simulink model "model_with_initial_conditions_v1"  (R2024b)
settings: Solver=VariableStepAuto  StartTime=0.0  StopTime=10.0  RelTol=1e-3
undefined symbols (not defined in the file): K1, K2, m
settings Model: Creator=njpan  LastModifiedBy=jacksonwright

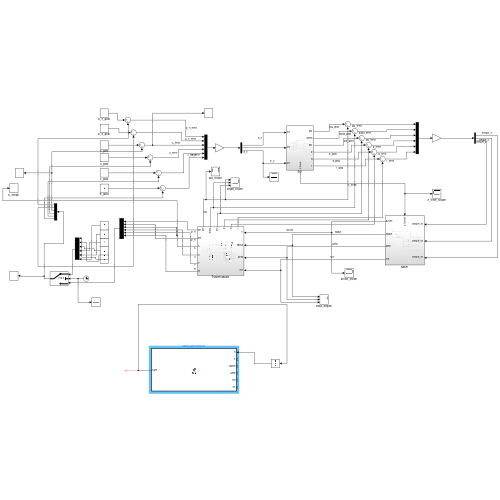
[thumbnail: Simulink's stored preview of the top-level diagram]
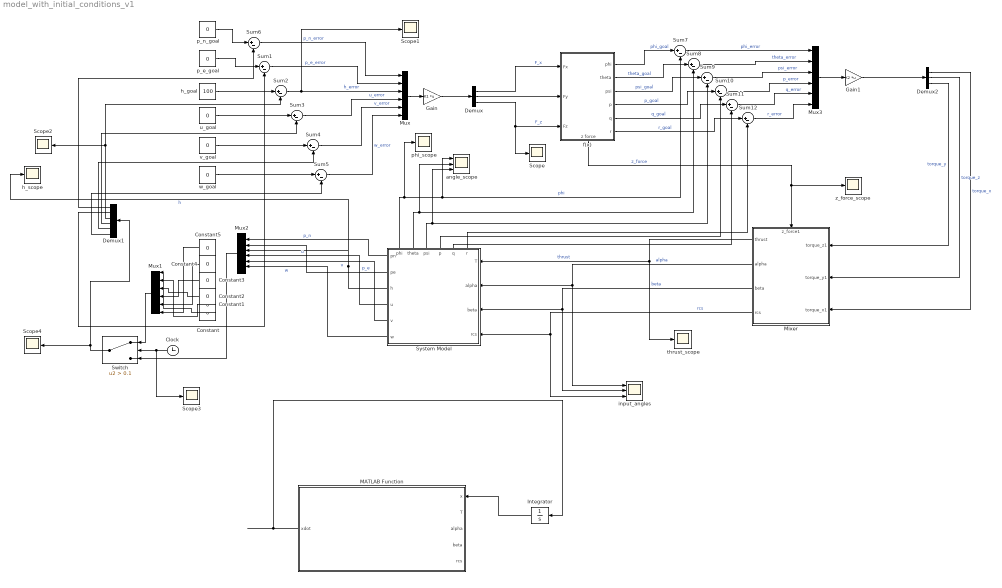
== system model_with_initial_conditions_v1 ==
  Clock : Clock
  Constant{,1..5} (6 alike) : Constant  Value=0
  Demux : Demux  Outputs=3
  Demux1 : Demux  Outputs=6
  Demux2 : Demux  Outputs=3
  Gain : Gain  Gain=K1  Multiplication=Matrix(K*u)
  Gain1 : Gain  Gain=K2  Multiplication=Matrix(K*u)
  Integrator : Integrator
  MATLAB Function : MATLAB Function  TreatAsAtomicUnit=on
  Mixer : Subsystem
      settings: PortSchema="{\"entries\":[{\"content\":{\"sides\":[{\"content\":{\"connectorIds\":[\"In1\",\"In2\",\"In3\"]},\"type\":\"ConnectorPlacement.EquallySpacedRectSide\",\"uuid\":\"e4ab6201-3171-425b-b678-f5a82ca77998\"},{\"content\":{\"connectorIds\":[\"Out1\",\"Out2\",\"Out3\",\"Out4\"],\"side\":\"RIGHT\"},\"type\":\"ConnectorPlacement.EquallySpacedRectSide\",\"uuid\":\"c6aae40c-8090-4a79-98d3-b60c0d3e66c5\"},{\"content\":{\"connectorIds\":[\"In4\"],\"side\":\"TOP\"},\"type\":\"ConnectorPlacement.EquallySpacedRectSide\",\"uuid\":\"89717ce5-f3d0-4b2e-8505-89723edf9773\"}]},\"type\":\"ConnectorPlacement.EquallySpacedConnector\",\"uuid\":\"ace876b5-bd23-4119-b1c7-2a296fd8fc0f\"}],\"packageUris\":[\"http://schema.mathworks.com/mf0/Connector/R2020b\"],\"version\":\"1.0\"}"
  Mux{,1..3} (4 alike) : Mux  Inputs=6
  Scope{,1..4} (5 alike) : Scope
  Sum{1..12} (12 alike) : Sum  Inputs=|+-
  Switch : Switch  Criteria=u2 > Threshold  Threshold=0.1  SaturateOnIntegerOverflow=off  InputSameDT=off
  System Model : Subsystem
      settings: PortSchema="{\"entries\":[{\"content\":{\"sides\":[{\"content\":{\"connectorIds\":[\"In1\",\"In2\",\"In3\",\"In4\"]},\"type\":\"ConnectorPlacement.EquallySpacedRectSide\",\"uuid\":\"8f145699-554a-4db3-b510-041d1b7c630e\"},{\"content\":{\"connectorIds\":[\"Out1\",\"Out2\",\"Out3\",\"Out4\",\"Out5\",\"Out6\"],\"side\":\"RIGHT\"},\"type\":\"ConnectorPlacement.EquallySpacedRectSide\",\"uuid\":\"6b085f61-d2ca-4739-902a-7b977a4f8bfa\"},{\"content\":{\"connectorIds\":[\"Out7\",\"Out8\",\"Out9\",\"Out10\",\"Out11\",\"Out12\"],\"side\":\"TOP\"},\"type\":\"ConnectorPlacement.EquallySpacedRectSide\",\"uuid\":\"4e3fe6dd-78f0-4e47-82e4-cad48dcfb91c\"}]},\"type\":\"ConnectorPlacement.EquallySpacedConnector\",\"uuid\":\"c7b0161a-0fea-43dd-8cee-87680deb6224\"}],\"packageUris\":[\"http://schema.mathworks.com/mf0/Connector/R2020b\"],\"version\":\"1.0\"}"
  angle_scope : Scope  NumInputPorts=3
  f(x) : Subsystem
      settings: PortSchema="{\"entries\":[{\"content\":{\"sides\":[{\"content\":{\"connectorIds\":[\"In1\",\"In2\",\"In3\"]},\"type\":\"ConnectorPlacement.EquallySpacedRectSide\",\"uuid\":\"e7aeffbb-634f-4153-9868-9d3e2e4280ad\"},{\"content\":{\"connectorIds\":[\"Out1\",\"Out2\",\"Out3\",\"Out4\",\"Out5\",\"Out6\"],\"side\":\"RIGHT\"},\"type\":\"ConnectorPlacement.EquallySpacedRectSide\",\"uuid\":\"e6d97028-2a10-4268-a5e2-55bbdc39a0c5\"},{\"content\":{\"side\":\"TOP\"},\"type\":\"ConnectorPlacement.EquallySpacedRectSide\",\"uuid\":\"fa716bc0-4a18-4661-a72d-62488d70bdc1\"},{\"content\":{\"connectorIds\":[\"Out7\"],\"side\":\"BOTTOM\"},\"type\":\"ConnectorPlacement.EquallySpacedRectSide\",\"uuid\":\"f442cf4b-5896-4629-a7d3-01e27d8da1cb\"}]},\"type\":\"ConnectorPlacement.EquallySpacedConnector\",\"uuid\":\"0a376c34-a895-4dfb-85c3-cafa4de2d877\"}],\"packageUris\":[\"http://schema.mathworks.com/mf0/Connector/R2020b\"],\"version\":\"1.0\"}"
  h_goal : Constant  Value=100
  h_scope : Scope
  input_angles : Scope  NumInputPorts=3
  p_e_goal : Constant  Value=0
  p_n_goal : Constant  Value=0
  phi_scope : Scope
  "thrust_scope " : Scope
  u_goal : Constant  Value=0
  v_goal : Constant  Value=0
  w_goal : Constant  Value=0
  z_force_scope : Scope
  wires:
  Sum6/1 -> Mux/1  "p_n_error"
  Sum1/1 -> Mux/2  "p_e_error"
  Sum2/1 -> Scope1/1, Mux/3  "h_error"
  Sum3/1 -> Mux/4  "u_error"
  Sum4/1 -> Mux/5  "v_error"
  Sum5/1 -> Mux/6  "w_error"
  System Model/1(pn) -> Mux2/1  "p_n"
  System Model/2(pe) -> Mux2/2  "p_e"
  System Model/3(h) -> h_scope/1, Mux2/3  "h"
  System Model/4(u) -> Mux2/4  "u"
  System Model/5(v) -> Mux2/5  "v"
  System Model/6(w) -> Mux2/6  "w"
  p_e_goal/1 -> Sum1/1
  h_goal/1 -> Sum2/1
  u_goal/1 -> Sum3/1
  v_goal/1 -> Sum4/1
  w_goal/1 -> Sum5/1
  Demux/3 -> f(x)/3(Fz), Scope/1  "F_z"
  p_n_goal/1 -> Sum6/1
  System Model/12(phi) -> angle_scope/1, Sum7/2, phi_scope/1  "phi"
  Sum7/1 -> Mux3/1  "phi_error"
  System Model/11(theta) -> angle_scope/2, Sum8/2
  Sum8/1 -> Mux3/2  "theta_error"
  System Model/10(psi) -> angle_scope/3, Sum9/2
  Sum9/1 -> Mux3/3  "psi_error"
  System Model/9(p) -> Sum10/2
  Sum10/1 -> Mux3/4  "p_error"
  System Model/8(q) -> Sum11/2
  Sum11/1 -> Mux3/5  "q_error"
  System Model/7(r) -> Sum12/2
  Sum12/1 -> Mux3/6  "r_error"
  Demux2/1 -> Mixer/3(torque_x1)  "torque_x"
  Demux2/3 -> Mixer/1(torque_z1)  "torque_y"
  Demux2/2 -> Mixer/2(torque_y1)  "torque_z"
  f(x)/7(z force) -> Mixer/4(z_force1), z_force_scope/1  "z_force"
  f(x)/6(r) -> Sum12/1  "r_goal"
  f(x)/5(q) -> Sum11/1  "q_goal"
  f(x)/4(p) -> Sum10/1  "p_goal"
  f(x)/3(psi) -> Sum9/1  "psi_goal"
  f(x)/2(theta) -> Sum8/1  "theta_goal"
  f(x)/1(phi) -> Sum7/1  "phi_goal"
  Mixer/4(rcs) -> input_angles/3, System Model/4(rcs)  "rcs"
  Mixer/3(beta) -> input_angles/2, System Model/3(beta)  "beta"
  Mixer/2(alpha) -> input_angles/1, System Model/2(alpha)  "alpha"
  Mixer/1(thrust) -> "thrust_scope "/1, System Model/1(T)  "thrust"
  Demux/1 -> f(x)/1(Fx)  "F_x"
  Gain/1 -> Demux/1
  Mux/1 -> Gain/1
  Demux/2 -> f(x)/2(Fy)
  Clock/1 -> Scope3/1, Switch/2
  Constant/1 -> Mux1/1
  Constant1/1 -> Mux1/2
  Constant2/1 -> Mux1/3
  Constant3/1 -> Mux1/4
  Constant4/1 -> Mux1/5
  Constant5/1 -> Mux1/6
  Mux1/1 -> Switch/1
  Switch/1 -> Scope4/1, Demux1/1
  Mux2/1 -> Switch/3
  Demux1/1 -> Sum6/2
  Demux1/2 -> Sum1/2
  Demux1/3 -> Sum2/2, Scope2/1
  Demux1/4 -> Sum3/2
  Demux1/5 -> Sum4/2
  Demux1/6 -> Sum5/2
  Mux3/1 -> Gain1/1
  Gain1/1 -> Demux2/1
  MATLAB Function/1(xdot) -> Integrator/1
  Integrator/1 -> MATLAB Function/1(x)

== system model_with_initial_conditions_v1/Mixer ==
  torque_z1 : Inport
  torque_y1 : Inport  Port=2
  torque_x1 : Inport  Port=3
  z_force1 : Inport  Port=4
  Divide : Product  Inputs=*/
  Divide1 : Product  Inputs=*/
  L : Constant
  LT_0 : Product
  Multiply : Gain  Gain=-1
  T_0 : Constant
  thrust : Outport
  alpha : Outport  Port=2
  beta : Outport  Port=3
  rcs : Outport  Port=4
  wires:
  torque_y1/1 -> Divide1/1
  Divide1/1 -> Multiply/1
  T_0/1 -> ?
  Divide/1 -> alpha/1
  L/1 -> LT_0/1
  LT_0/1 -> Divide1/2, Divide/2
  torque_z1/1 -> rcs/1
  z_force1/1 -> LT_0/2, thrust/1
  Multiply/1 -> beta/1
  torque_x1/1 -> Divide/1

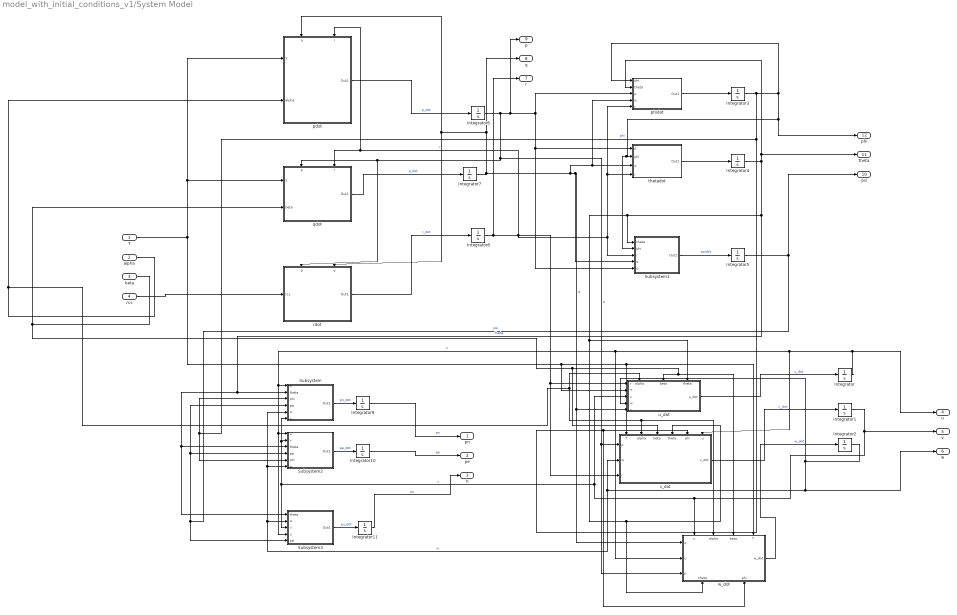
== system model_with_initial_conditions_v1/System Model ==
  T : Inport
  alpha : Inport  Port=2
  beta : Inport  Port=3
  rcs : Inport  Port=4
  Integrator{,1..11} (12 alike) : Integrator
  Subsystem : Subsystem
  Subsystem1 : Subsystem
  Subsystem2 : Subsystem
  Subsystem3 : Subsystem
  pdot : Subsystem
      settings: PortSchema="{\"entries\":[{\"content\":{\"sides\":[{\"content\":{\"connectorIds\":[\"In1\",\"In2\"]},\"type\":\"ConnectorPlacement.EquallySpacedRectSide\",\"uuid\":\"6ab7a4db-f82d-4cec-b306-dad3d39631b0\"},{\"content\":{\"connectorIds\":[\"Out1\"],\"side\":\"RIGHT\"},\"type\":\"ConnectorPlacement.EquallySpacedRectSide\",\"uuid\":\"9acc64a4-ce2e-4f5d-b63d-5066b3292dd6\"},{\"content\":{\"connectorIds\":[\"In3\",\"In4\"],\"side\":\"TOP\"},\"type\":\"ConnectorPlacement.EquallySpacedRectSide\",\"uuid\":\"997ab406-422d-44bc-a1c0-6727b241ac30\"}]},\"type\":\"ConnectorPlacement.EquallySpacedConnector\",\"uuid\":\"7642bc88-cdbb-4c52-8569-24becb616f7b\"}],\"packageUris\":[\"http://schema.mathworks.com/mf0/Connector/R2020b\"],\"version\":\"1.0\"}"
  phidot : Subsystem
  qdot : Subsystem
      settings: PortSchema="{\"entries\":[{\"content\":{\"sides\":[{\"content\":{\"connectorIds\":[\"In1\",\"In2\"]},\"type\":\"ConnectorPlacement.EquallySpacedRectSide\",\"uuid\":\"6ab7a4db-f82d-4cec-b306-dad3d39631b0\"},{\"content\":{\"connectorIds\":[\"Out1\"],\"side\":\"RIGHT\"},\"type\":\"ConnectorPlacement.EquallySpacedRectSide\",\"uuid\":\"9acc64a4-ce2e-4f5d-b63d-5066b3292dd6\"},{\"content\":{\"connectorIds\":[\"In3\",\"In4\"],\"side\":\"TOP\"},\"type\":\"ConnectorPlacement.EquallySpacedRectSide\",\"uuid\":\"997ab406-422d-44bc-a1c0-6727b241ac30\"}]},\"type\":\"ConnectorPlacement.EquallySpacedConnector\",\"uuid\":\"7642bc88-cdbb-4c52-8569-24becb616f7b\"}],\"packageUris\":[\"http://schema.mathworks.com/mf0/Connector/R2020b\"],\"version\":\"1.0\"}"
  rdot : Subsystem
      settings: PortSchema="{\"entries\":[{\"content\":{\"sides\":[{\"content\":{\"connectorIds\":[\"In1\"]},\"type\":\"ConnectorPlacement.EquallySpacedRectSide\",\"uuid\":\"6ab7a4db-f82d-4cec-b306-dad3d39631b0\"},{\"content\":{\"connectorIds\":[\"Out1\"],\"side\":\"RIGHT\"},\"type\":\"ConnectorPlacement.EquallySpacedRectSide\",\"uuid\":\"9acc64a4-ce2e-4f5d-b63d-5066b3292dd6\"},{\"content\":{\"connectorIds\":[\"In2\",\"In3\"],\"side\":\"TOP\"},\"type\":\"ConnectorPlacement.EquallySpacedRectSide\",\"uuid\":\"997ab406-422d-44bc-a1c0-6727b241ac30\"}]},\"type\":\"ConnectorPlacement.EquallySpacedConnector\",\"uuid\":\"7642bc88-cdbb-4c52-8569-24becb616f7b\"}],\"packageUris\":[\"http://schema.mathworks.com/mf0/Connector/R2020b\"],\"version\":\"1.0\"}"
  thetadot : Subsystem
  u_dot : Subsystem
      settings: PortSchema="{\"entries\":[{\"content\":{\"sides\":[{\"content\":{\"connectorIds\":[\"In1\",\"In2\",\"In3\",\"In4\",\"In5\"]},\"type\":\"ConnectorPlacement.EquallySpacedRectSide\",\"uuid\":\"64eef309-b73c-48da-be96-ce790931dba8\"},{\"content\":{\"connectorIds\":[\"Out1\"],\"side\":\"RIGHT\"},\"type\":\"ConnectorPlacement.EquallySpacedRectSide\",\"uuid\":\"ffd61837-7847-4a6b-9743-1cbc97c13cef\"},{\"content\":{\"connectorIds\":[\"In6\",\"In7\",\"In8\"],\"side\":\"TOP\"},\"type\":\"ConnectorPlacement.EquallySpacedRectSide\",\"uuid\":\"abc28f87-1872-4f5b-8dd3-d7626c998f10\"}]},\"type\":\"ConnectorPlacement.EquallySpacedConnector\",\"uuid\":\"8e3aaafe-c778-4166-b859-e0c398154b98\"}],\"packageUris\":[\"http://schema.mathworks.com/mf0/Connector/R2020b\"],\"version\":\"1.0\"}"
  v_dot : Subsystem
      settings: PortSchema="{\"entries\":[{\"content\":{\"sides\":[{\"content\":{\"connectorIds\":[\"In1\",\"In2\",\"In3\"]},\"type\":\"ConnectorPlacement.EquallySpacedRectSide\",\"uuid\":\"a4e0a5eb-8103-4107-8c28-a650b6e2a478\"},{\"content\":{\"connectorIds\":[\"Out1\"],\"side\":\"RIGHT\"},\"type\":\"ConnectorPlacement.EquallySpacedRectSide\",\"uuid\":\"35fa197a-615e-40cd-8bc5-f0655a9643f8\"},{\"content\":{\"connectorIds\":[\"In4\",\"In5\",\"In6\",\"In7\",\"In8\",\"In9\"],\"side\":\"TOP\"},\"type\":\"ConnectorPlacement.EquallySpacedRectSide\",\"uuid\":\"13c066ef-0cad-42db-9278-8f4c2c4533fa\"},{\"content\":{\"side\":\"BOTTOM\"},\"type\":\"ConnectorPlacement.EquallySpacedRectSide\",\"uuid\":\"cb84b247-9b09-4767-abf0-36c3b728ef40\"}]},\"type\":\"ConnectorPlacement.EquallySpacedConnector\",\"uuid\":\"cd4e31bf-f144-43ed-bb49-bc1ff9ad93b8\"}],\"packageUris\":[\"http://schema.mathworks.com/mf0/Connector/R2020b\"],\"version\":\"1.0\"}"
  w_dot : Subsystem
      settings: PortSchema="{\"entries\":[{\"content\":{\"sides\":[{\"content\":{\"connectorIds\":[\"In1\",\"In2\",\"In3\"]},\"type\":\"ConnectorPlacement.EquallySpacedRectSide\",\"uuid\":\"a4e0a5eb-8103-4107-8c28-a650b6e2a478\"},{\"content\":{\"connectorIds\":[\"Out1\"],\"side\":\"RIGHT\"},\"type\":\"ConnectorPlacement.EquallySpacedRectSide\",\"uuid\":\"35fa197a-615e-40cd-8bc5-f0655a9643f8\"},{\"content\":{\"connectorIds\":[\"In4\",\"In5\",\"In6\",\"In7\"],\"side\":\"TOP\"},\"type\":\"ConnectorPlacement.EquallySpacedRectSide\",\"uuid\":\"13c066ef-0cad-42db-9278-8f4c2c4533fa\"},{\"content\":{\"connectorIds\":[\"In8\",\"In9\"],\"side\":\"BOTTOM\"},\"type\":\"ConnectorPlacement.EquallySpacedRectSide\",\"uuid\":\"051f7a09-e622-45d9-8710-37c092191ba7\"}]},\"type\":\"ConnectorPlacement.EquallySpacedConnector\",\"uuid\":\"cd4e31bf-f144-43ed-bb49-bc1ff9ad93b8\"}],\"packageUris\":[\"http://schema.mathworks.com/mf0/Connector/R2020b\"],\"version\":\"1.0\"}"
  pn : Outport
  pe : Outport  Port=2
  h : Outport  Port=3
  u : Outport  Port=4
  v : Outport  Port=5
  w : Outport  Port=6
  r : Outport  Port=7
  q : Outport  Port=8
  p : Outport  Port=9
  psi : Outport  Port=10
  theta : Outport  Port=11
  phi : Outport  Port=12
  wires:
  Integrator11/1 -> h/1  "pu"
  pdot/1(Out1) -> Integrator6/1  "p_dot"
  Integrator8/1 -> r/1, v_dot/3(r), u_dot/1(r), thetadot/4(r), phidot/5(r), Subsystem1/3(r), qdot/4(r), pdot/4(r)  "r"
  qdot/1(Out1) -> Integrator7/1  "q_dot"
  Subsystem1/1(Out1) -> Integrator5/1  "psidot"
  Integrator1/1 -> v/1, Subsystem2/2(v), Subsystem/6(v), Subsystem3/3(v), u_dot/3(v), w_dot/4(v)  "v"
  beta/1 -> u_dot/7(beta), w_dot/6(beta), v_dot/6(beta), qdot/2(beta)
  w_dot/1(w_dot) -> Integrator2/1  "w_dot"
  alpha/1 -> v_dot/5(alpha), w_dot/5(alpha), u_dot/6(alpha), pdot/2(alpha)
  T/1 -> v_dot/4(T), w_dot/7(T), u_dot/2(T), pdot/1(T), qdot/1(T)
  Subsystem3/1(Out1) -> Integrator11/1  "pu_dot"
  Subsystem/1(Out1) -> Integrator9/1  "pn_dot"
  Integrator4/1 -> Subsystem3/1(theta), Subsystem2/3(theta), Subsystem/2(theta), v_dot/7(theta), w_dot/8(theta), u_dot/8(theta), Subsystem1/1(theta), phidot/2(theta), theta/1  "theta"
  Integrator10/1 -> pe/1  "pe"
  Integrator5/1 -> psi/1, Subsystem/4(psi), Subsystem2/4(psi), Subsystem3/5(psi)  "psi"
  Integrator9/1 -> pn/1  "pn"
  Integrator2/1 -> Subsystem/5(w), Subsystem2/6(w), Subsystem3/2(w), v_dot/2(w), w/1, u_dot/4(w)  "w"
  Integrator7/1 -> q/1, pdot/3(q), rdot/3(q), w_dot/1(q), u_dot/5(q), Subsystem1/4(q), phidot/4(q), thetadot/3(q)  "q"
  rdot/1(Out1) -> Integrator8/1  "r_dot"
  rcs/1 -> rdot/1(rcs)
  u_dot/1(u_dot) -> Integrator/1  "u_dot"
  Integrator/1 -> u/1, v_dot/9(u), Subsystem3/4(u), Subsystem2/1(u), Subsystem/1(u), w_dot/2(u)  "u"
  thetadot/1(Out1) -> Integrator4/1
  Subsystem2/1(Out1) -> Integrator10/1  "pe_dot"
  Integrator3/1 -> Subsystem2/5(phi), Subsystem/3(phi), w_dot/9(phi), v_dot/8(phi), phi/1, Subsystem1/2(phi), thetadot/2(phi), phidot/1(phi)  "phi"
  v_dot/1(v_dot) -> Integrator1/1  "v_dot"
  phidot/1(Out1) -> Integrator3/1
  Integrator6/1 -> p/1, Subsystem1/5(p), thetadot/1(p), phidot/3(p), w_dot/3(p), v_dot/1(p), rdot/2(p), qdot/3(p)  "p"

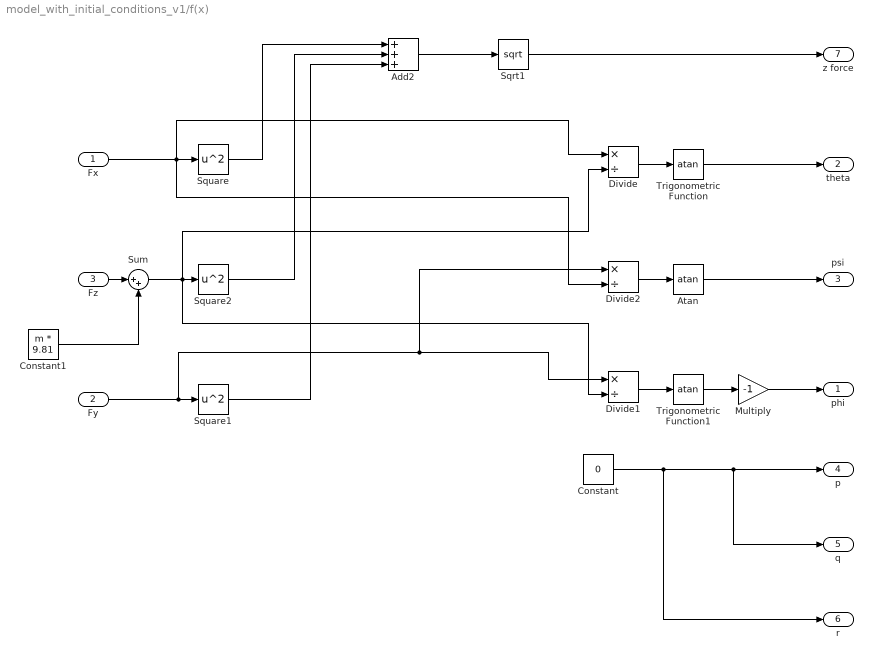
== system model_with_initial_conditions_v1/f(x) ==
  Fx : Inport
  Fy : Inport  Port=2
  Fz : Inport  Port=3
  Add2 : Sum  Inputs=+++
  Atan : Trigonometry  Operator=atan
  Constant : Constant  Value=0
  Constant1 : Constant  Value=m * 9.81
  Divide : Product  Inputs=*/
  Divide1 : Product  Inputs=*/
  Divide2 : Product  Inputs=*/
  Multiply : Gain  Gain=-1
  Sqrt1 : Sqrt
  Square : Math  Operator=square
  Square1 : Math  Operator=square
  Square2 : Math  Operator=square
  Sum : Sum  Inputs=|++
  Trigonometric Function : Trigonometry  Operator=atan
  Trigonometric Function1 : Trigonometry  Operator=atan
  phi : Outport
  theta : Outport  Port=2
  psi : Outport  Port=3
  p : Outport  Port=4
  q : Outport  Port=5
  r : Outport  Port=6
  z force : Outport  Port=7
  wires:
  Multiply/1 -> phi/1
  Divide/1 -> Trigonometric Function/1
  Square1/1 -> Add2/3
  Square/1 -> Add2/1
  Divide1/1 -> Trigonometric Function1/1
  Fx/1 -> Divide/1, Divide2/2, Square/1
  Atan/1 -> psi/1
  Add2/1 -> Sqrt1/1
  Square2/1 -> Add2/2
  Fy/1 -> Divide2/1, Divide1/1, Square1/1
  Divide2/1 -> Atan/1
  Trigonometric Function/1 -> theta/1
  Sqrt1/1 -> z force/1
  Constant/1 -> r/1, q/1, p/1
  Trigonometric Function1/1 -> Multiply/1
  Sum/1 -> Divide1/2, Divide/2, Square2/1
  Fz/1 -> Sum/1
  Constant1/1 -> Sum/2

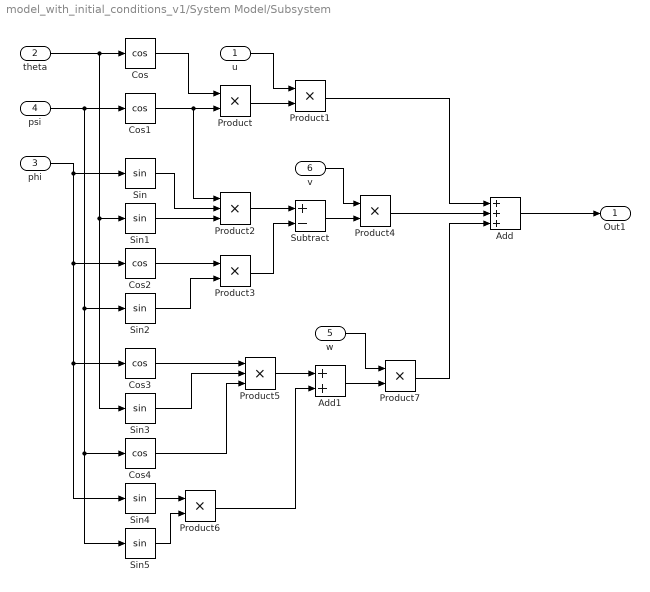
== system model_with_initial_conditions_v1/System Model/Subsystem ==
  u : Inport
  theta : Inport  Port=2
  phi : Inport  Port=3
  psi : Inport  Port=4
  w : Inport  Port=5
  v : Inport  Port=6
  Add : Sum  Inputs=+++
  Add1 : Sum
  Cos{,1..4} (5 alike) : Trigonometry  Operator=cos
  Product{,1,3..4,6..7} (6 alike) : Product
  Product2 : Product  Inputs=3
  Product5 : Product  Inputs=3
  Sin{,1..5} (6 alike) : Trigonometry
  Subtract : Sum  Inputs=+-
  Out1 : Outport
  wires:
  theta/1 -> Sin3/1, Sin1/1, Cos/1
  psi/1 -> Sin5/1, Cos4/1, Sin2/1, Cos1/1
  Cos1/1 -> Product2/1, Product/2
  Cos/1 -> Product/1
  Product/1 -> Product1/2
  u/1 -> Product1/1
  Product1/1 -> Add/1
  Add/1 -> Out1/1
  phi/1 -> Sin4/1, Cos3/1, Cos2/1, Sin/1
  Sin1/1 -> Product2/3
  Sin/1 -> Product2/2
  Product2/1 -> Subtract/1
  Cos2/1 -> Product3/1
  Sin2/1 -> Product3/2
  Product3/1 -> Subtract/2
  Subtract/1 -> Product4/2
  v/1 -> Product4/1
  Product4/1 -> Add/2
  Cos3/1 -> Product5/1
  Sin3/1 -> Product5/2
  Cos4/1 -> Product5/3
  Product5/1 -> Add1/1
  Sin4/1 -> Product6/1
  Sin5/1 -> Product6/2
  Product6/1 -> Add1/2
  Add1/1 -> Product7/2
  w/1 -> Product7/1
  Product7/1 -> Add/3

== system model_with_initial_conditions_v1/System Model/Subsystem1 ==
  theta : Inport
  phi : Inport  Port=2
  r : Inport  Port=3
  q : Inport  Port=4
  p : Inport  Port=5
  Add : Sum  Inputs=+++
  Constant : Constant  Value=0
  Cos : Trigonometry  Operator=cos
  Cos1 : Trigonometry  Operator=cos
  Divide : Product  Inputs=*/
  Divide1 : Product  Inputs=*/
  Product : Product
  Product1 : Product
  Product2 : Product
  Sin : Trigonometry
  Out1 : Outport
  wires:
  phi/1 -> Cos1/1, Sin/1
  theta/1 -> Cos/1
  Sin/1 -> Divide/1
  Divide/1 -> Product/2
  q/1 -> Product/1
  Constant/1 -> Product1/2
  p/1 -> Product1/1
  Product/1 -> Add/2
  Product1/1 -> Add/1
  Add/1 -> Out1/1
  Cos1/1 -> Divide1/1
  Cos/1 -> Divide1/2, Divide/2
  r/1 -> Product2/1
  Divide1/1 -> Product2/2
  Product2/1 -> Add/3

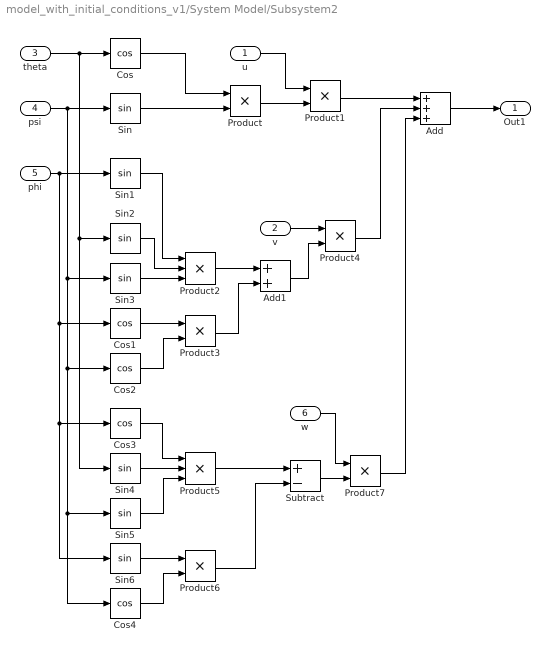
== system model_with_initial_conditions_v1/System Model/Subsystem2 ==
  u : Inport
  v : Inport  Port=2
  theta : Inport  Port=3
  psi : Inport  Port=4
  phi : Inport  Port=5
  w : Inport  Port=6
  Add : Sum  Inputs=+++
  Add1 : Sum
  Cos{,1..4} (5 alike) : Trigonometry  Operator=cos
  Product{,1,3..4,6..7} (6 alike) : Product
  Product2 : Product  Inputs=3
  Product5 : Product  Inputs=3
  Sin{,1..6} (7 alike) : Trigonometry
  Subtract : Sum  Inputs=+-
  Out1 : Outport
  wires:
  theta/1 -> Sin4/1, Sin2/1, Cos/1
  psi/1 -> Cos4/1, Sin5/1, Cos2/1, Sin3/1, Sin/1
  Sin/1 -> Product/2
  Cos/1 -> Product/1
  Product/1 -> Product1/2
  u/1 -> Product1/1
  Product1/1 -> Add/1
  phi/1 -> Sin6/1, Cos3/1, Cos1/1, Sin1/1
  Sin3/1 -> Product2/3
  Sin2/1 -> Product2/2
  Sin1/1 -> Product2/1
  Cos1/1 -> Product3/1
  Cos2/1 -> Product3/2
  Product2/1 -> Add1/1
  Product3/1 -> Add1/2
  v/1 -> Product4/1
  Add1/1 -> Product4/2
  Product4/1 -> Add/2
  Add/1 -> Out1/1
  Cos3/1 -> Product5/1
  Sin4/1 -> Product5/2
  Sin5/1 -> Product5/3
  Product5/1 -> Subtract/1
  Sin6/1 -> Product6/1
  Product6/1 -> Subtract/2
  Cos4/1 -> Product6/2
  Subtract/1 -> Product7/2
  w/1 -> Product7/1
  Product7/1 -> Add/3

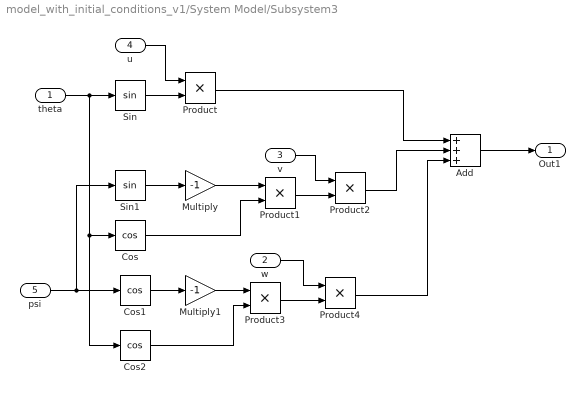
== system model_with_initial_conditions_v1/System Model/Subsystem3 ==
  theta : Inport
  w : Inport  Port=2
  v : Inport  Port=3
  u : Inport  Port=4
  psi : Inport  Port=5
  Add : Sum  Inputs=+++
  Cos : Trigonometry  Operator=cos
  Cos1 : Trigonometry  Operator=cos
  Cos2 : Trigonometry  Operator=cos
  Multiply : Gain  Gain=-1
  Multiply1 : Gain  Gain=-1
  Product{,1..4} (5 alike) : Product
  Sin : Trigonometry
  Sin1 : Trigonometry
  Out1 : Outport
  wires:
  Add/1 -> Out1/1
  theta/1 -> Cos2/1, Cos/1, Sin/1
  Sin/1 -> Product/2
  u/1 -> Product/1
  Product/1 -> Add/1
  psi/1 -> Sin1/1, Cos1/1
  Sin1/1 -> Multiply/1
  Multiply/1 -> Product1/1
  Cos/1 -> Product1/2
  Product1/1 -> Product2/2
  v/1 -> Product2/1
  Product2/1 -> Add/2
  Cos1/1 -> Multiply1/1
  Multiply1/1 -> Product3/1
  Cos2/1 -> Product3/2
  Product3/1 -> Product4/2
  w/1 -> Product4/1
  Product4/1 -> Add/3

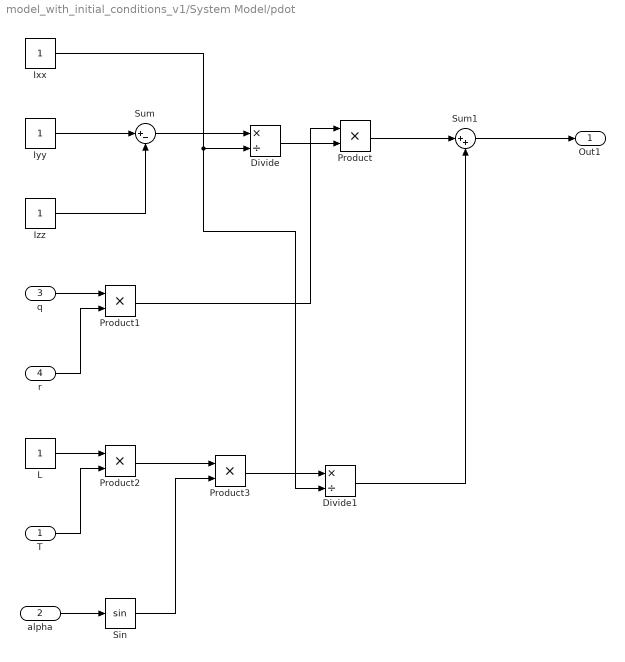
== system model_with_initial_conditions_v1/System Model/pdot ==
  T : Inport
  alpha : Inport  Port=2
  q : Inport  Port=3
  r : Inport  Port=4
  Divide : Product  Inputs=*/
  Divide1 : Product  Inputs=*/
  Ixx : Constant
  Iyy : Constant
  Izz : Constant
  L : Constant
  Product{,1..3} (4 alike) : Product
  Sin : Trigonometry
  Sum : Sum  Inputs=|+-
  Sum1 : Sum  Inputs=|++
  Out1 : Outport
  wires:
  Iyy/1 -> Sum/1
  Izz/1 -> Sum/2
  Sum/1 -> Divide/1
  Ixx/1 -> Divide1/2, Divide/2
  Divide/1 -> Product/2
  q/1 -> Product1/1
  r/1 -> Product1/2
  Product1/1 -> Product/1
  L/1 -> Product2/1
  T/1 -> Product2/2
  alpha/1 -> Sin/1
  Product2/1 -> Product3/1
  Sin/1 -> Product3/2
  Product3/1 -> Divide1/1
  Product/1 -> Sum1/1
  Divide1/1 -> Sum1/2
  Sum1/1 -> Out1/1

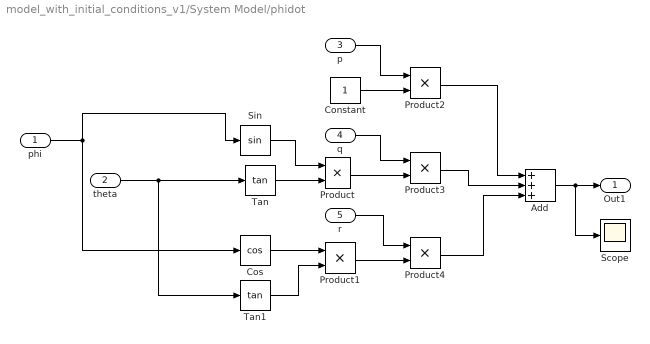
== system model_with_initial_conditions_v1/System Model/phidot ==
  phi : Inport
  theta : Inport  Port=2
  p : Inport  Port=3
  q : Inport  Port=4
  r : Inport  Port=5
  Add : Sum  Inputs=+++
  Constant : Constant
  Cos : Trigonometry  Operator=cos
  Product{,1..4} (5 alike) : Product
  Scope : Scope
  Sin : Trigonometry
  Tan : Trigonometry  Operator=tan
  Tan1 : Trigonometry  Operator=tan
  Out1 : Outport
  wires:
  theta/1 -> Tan1/1, Tan/1
  phi/1 -> Cos/1, Sin/1
  Sin/1 -> Product/1
  Tan/1 -> Product/2
  Cos/1 -> Product1/1
  Tan1/1 -> Product1/2
  Constant/1 -> Product2/2
  p/1 -> Product2/1
  Product/1 -> Product3/2
  q/1 -> Product3/1
  Product1/1 -> Product4/2
  r/1 -> Product4/1
  Product2/1 -> Add/1
  Product3/1 -> Add/2
  Product4/1 -> Add/3
  Add/1 -> Scope/1, Out1/1

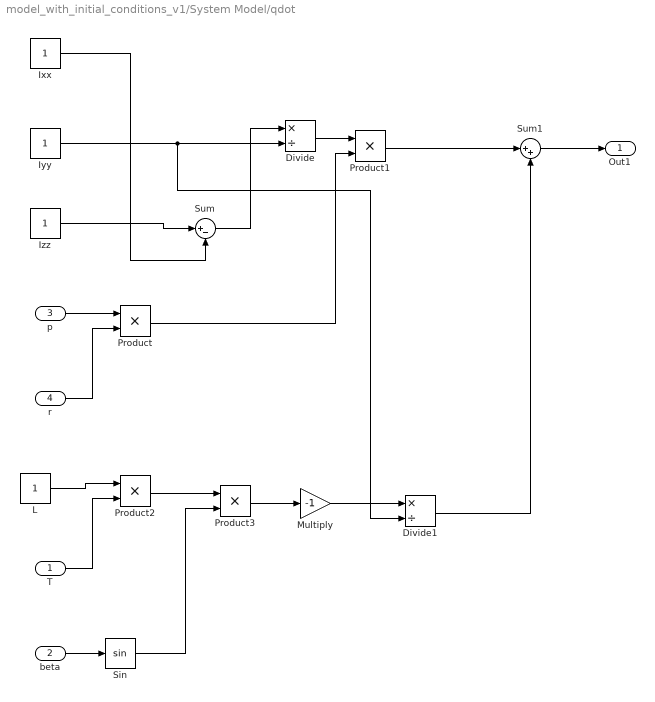
== system model_with_initial_conditions_v1/System Model/qdot ==
  T : Inport
  beta : Inport  Port=2
  p : Inport  Port=3
  r : Inport  Port=4
  Divide : Product  Inputs=*/
  Divide1 : Product  Inputs=*/
  Ixx : Constant
  Iyy : Constant
  Izz : Constant
  L : Constant
  Multiply : Gain  Gain=-1
  Product{,1..3} (4 alike) : Product
  Sin : Trigonometry
  Sum : Sum  Inputs=|+-
  Sum1 : Sum  Inputs=|++
  Out1 : Outport
  wires:
  Izz/1 -> Sum/1
  Ixx/1 -> Sum/2
  Iyy/1 -> Divide1/2, Divide/2
  Sum/1 -> Divide/1
  p/1 -> Product/1
  r/1 -> Product/2
  Divide/1 -> Product1/1
  Product/1 -> Product1/2
  L/1 -> Product2/1
  T/1 -> Product2/2
  beta/1 -> Sin/1
  Product2/1 -> Product3/1
  Sin/1 -> Product3/2
  Product3/1 -> Multiply/1
  Multiply/1 -> Divide1/1
  Product1/1 -> Sum1/1
  Divide1/1 -> Sum1/2
  Sum1/1 -> Out1/1

== system model_with_initial_conditions_v1/System Model/rdot ==
  rcs : Inport
  p : Inport  Port=2
  q : Inport  Port=3
  Divide : Product  Inputs=*/
  Divide1 : Product  Inputs=*/
  Ixx : Constant
  Iyy : Constant
  Izz : Constant
  Product : Product
  Product1 : Product
  Sum : Sum  Inputs=|+-
  Sum1 : Sum  Inputs=|++
  Out1 : Outport
  wires:
  Ixx/1 -> Sum/1
  Sum/1 -> Divide/1
  Izz/1 -> Divide1/2, Divide/2
  p/1 -> Product/1
  q/1 -> Product/2
  Divide/1 -> Product1/1
  Product/1 -> Product1/2
  rcs/1 -> Divide1/1
  Product1/1 -> Sum1/1
  Divide1/1 -> Sum1/2
  Sum1/1 -> Out1/1
  Iyy/1 -> Sum/2

== system model_with_initial_conditions_v1/System Model/thetadot ==
  p : Inport
  phi : Inport  Port=2
  q : Inport  Port=3
  r : Inport  Port=4
  Add : Sum  Inputs=++-
  Constant : Constant  Value=0
  Cos : Trigonometry  Operator=cos
  Product : Product
  Product1 : Product
  Product2 : Product
  Scope : Scope
  Sin : Trigonometry
  Out1 : Outport
  wires:
  phi/1 -> Cos/1, Sin/1
  Sin/1 -> Product/2
  r/1 -> Product/1
  Cos/1 -> Product1/2
  q/1 -> Product1/1
  Constant/1 -> Product2/2
  p/1 -> Product2/1
  Product2/1 -> Add/1
  Product1/1 -> Add/2
  Product/1 -> Add/3
  Add/1 -> Scope/1, Out1/1

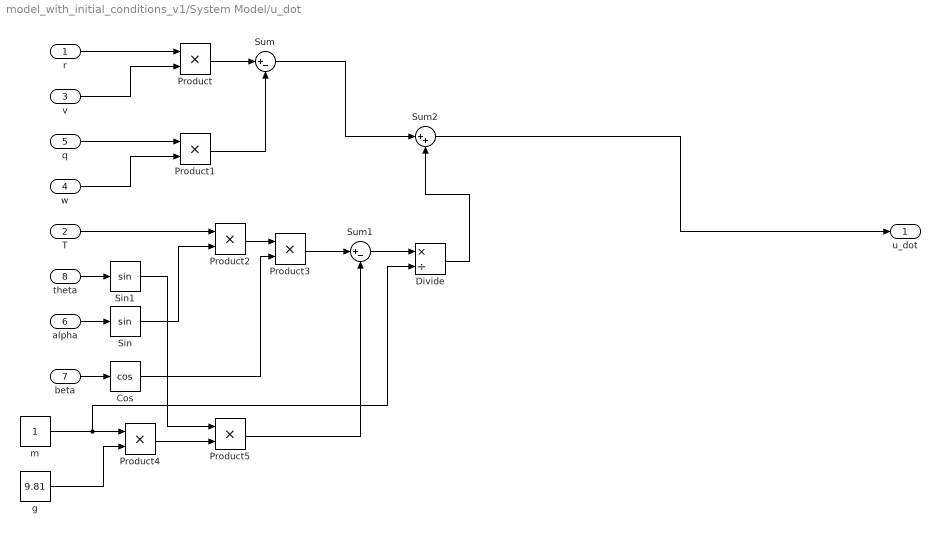
== system model_with_initial_conditions_v1/System Model/u_dot ==
  r : Inport
  T : Inport  Port=2
  v : Inport  Port=3
  w : Inport  Port=4
  q : Inport  Port=5
  alpha : Inport  Port=6
  beta : Inport  Port=7
  theta : Inport  Port=8
  Cos : Trigonometry  Operator=cos
  Divide : Product  Inputs=*/
  Product{,1..5} (6 alike) : Product
  Sin : Trigonometry
  Sin1 : Trigonometry
  Sum : Sum  Inputs=|+-
  Sum1 : Sum  Inputs=|+-
  Sum2 : Sum  Inputs=|++
  g : Constant  Value=9.81
  m : Constant
  u_dot : Outport
  wires:
  Sum2/1 -> u_dot/1
  r/1 -> Product/1
  v/1 -> Product/2
  q/1 -> Product1/1
  w/1 -> Product1/2
  Product/1 -> Sum/1
  Product1/1 -> Sum/2
  alpha/1 -> Sin/1
  beta/1 -> Cos/1
  theta/1 -> Sin1/1
  T/1 -> Product2/1
  Sin/1 -> Product2/2
  Cos/1 -> Product3/2
  Product2/1 -> Product3/1
  m/1 -> Divide/2, Product4/1
  g/1 -> Product4/2
  Product4/1 -> Product5/2
  Sin1/1 -> Product5/1
  Product3/1 -> Sum1/1
  Product5/1 -> Sum1/2
  Sum1/1 -> Divide/1
  Sum/1 -> Sum2/1
  Divide/1 -> Sum2/2

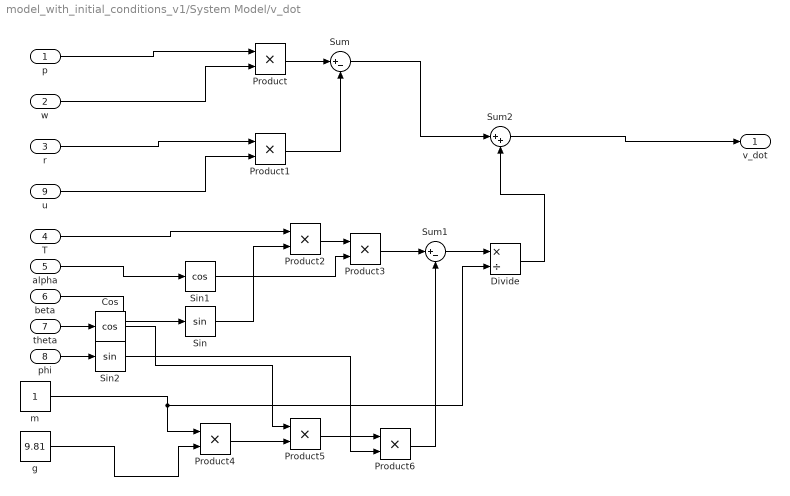
== system model_with_initial_conditions_v1/System Model/v_dot ==
  p : Inport
  w : Inport  Port=2
  r : Inport  Port=3
  T : Inport  Port=4
  alpha : Inport  Port=5
  beta : Inport  Port=6
  theta : Inport  Port=7
  phi : Inport  Port=8
  u : Inport  Port=9
  Cos : Trigonometry  Operator=cos
  Divide : Product  Inputs=*/
  Product{,1..6} (7 alike) : Product
  Sin : Trigonometry
  Sin1 : Trigonometry  Operator=cos
  Sin2 : Trigonometry
  Sum : Sum  Inputs=|+-
  Sum1 : Sum  Inputs=|+-
  Sum2 : Sum  Inputs=|++
  g : Constant  Value=9.81
  m : Constant
  v_dot : Outport
  wires:
  Product1/1 -> Sum/2
  p/1 -> Product/1
  r/1 -> Product1/1
  w/1 -> Product/2
  u/1 -> Product1/2
  Product/1 -> Sum/1
  beta/1 -> Sin/1
  Sin/1 -> Product2/2
  Divide/1 -> Sum2/2
  alpha/1 -> Sin1/1
  Sum1/1 -> Divide/1
  g/1 -> Product4/2
  Sum/1 -> Sum2/1
  Product3/1 -> Sum1/1
  theta/1 -> Cos/1
  Product4/1 -> Product5/2
  Product2/1 -> Product3/1
  m/1 -> Product4/1, Divide/2
  Sum2/1 -> v_dot/1
  T/1 -> Product2/1
  Sin1/1 -> Product3/2
  phi/1 -> Sin2/1
  Cos/1 -> Product5/1
  Product5/1 -> Product6/1
  Sin2/1 -> Product6/2
  Product6/1 -> Sum1/2

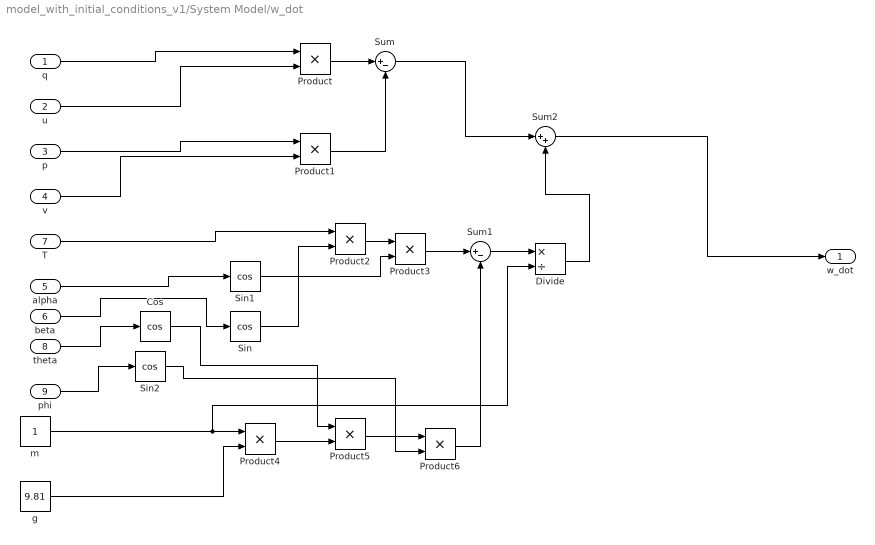
== system model_with_initial_conditions_v1/System Model/w_dot ==
  q : Inport
  u : Inport  Port=2
  p : Inport  Port=3
  v : Inport  Port=4
  alpha : Inport  Port=5
  beta : Inport  Port=6
  T : Inport  Port=7
  theta : Inport  Port=8
  phi : Inport  Port=9
  Cos : Trigonometry  Operator=cos
  Divide : Product  Inputs=*/
  Product{,1..6} (7 alike) : Product
  Sin : Trigonometry  Operator=cos
  Sin1 : Trigonometry  Operator=cos
  Sin2 : Trigonometry  Operator=cos
  Sum : Sum  Inputs=|+-
  Sum1 : Sum  Inputs=|+-
  Sum2 : Sum  Inputs=|++
  g : Constant  Value=9.81
  m : Constant
  w_dot : Outport
  wires:
  alpha/1 -> Sin1/1
  Cos/1 -> Product5/1
  p/1 -> Product1/1
  m/1 -> Divide/2, Product4/1
  q/1 -> Product/1
  Product2/1 -> Product3/1
  Product3/1 -> Sum1/1
  Product4/1 -> Product5/2
  Sum/1 -> Sum2/1
  Product/1 -> Sum/1
  Divide/1 -> Sum2/2
  Sum1/1 -> Divide/1
  Sin/1 -> Product2/2
  Product1/1 -> Sum/2
  Sum2/1 -> w_dot/1
  beta/1 -> Sin/1
  g/1 -> Product4/2
  u/1 -> Product/2
  v/1 -> Product1/2
  Product5/1 -> Product6/1
  Product6/1 -> Sum1/2
  Sin1/1 -> Product3/2
  Sin2/1 -> Product6/2
  T/1 -> Product2/1
  theta/1 -> Cos/1
  phi/1 -> Sin2/1

== matlab function model_with_initial_conditions_v1/MATLAB Function ==
  data: x input; T input; xdot output; alpha input; beta input; rcs input
function xdot = fcn(x, T, alpha, beta, rcs)

m = 1;
g = 9.81;
L = 1;
Ixx = 1;
Iyy = 1;
Izz = 1;

% pn = x(1);
% pe = x(2);
% pu = x(3);
u = x(4);
v = x(5);
w = x(6);
phi = x(7);
theta = x(8);
psi = x(9);
p = x(10);
q = x(11);
r = x(12);

xdot = [];

xdot(1) = cos(theta)*cost(psi)*u + (sin(phi)*sin(theta)*cos(psi) - cos(phi)*sin(psi))*v + (cos(phi)*sin(theta)*cos(psi)+sin(phi)*sin(psi))*w;
xdot(2) = cos(theta)*sin(psi)*u + (sin(phi)*sin(theta)*sin(psi)+cos(phi)*cos(psi))*v + (cos(phi)*sin(theta)*sin(psi)-sin(phi)*cos(psi))*w;
xdot(3) = sin(theta)*u - sin(phi)*cos(theta)*v - cos(phi)*cos(theta)*w;
xdot(4) = r*v - q*w + (T*sin(alpha)*cos(beta) - m*g*sin(theta))/m;
xdot(5) = p*w - r*u + (T*sin(beta)*cos(alpha) - m*g*cos(theta)*sin(phi))/m;
xdot(6) = q*u - p*v + (T*cos(alpha)*cos(beta) - m*g*cos(theta)*cos(phi))/m;
xdot(7) = p + sin(phi)*tan(theta)*q + cos(phi)*tan(theta)*r;
xdot(8) = cos(phi)*q - sin(phi)*r;
xdot(9) = sin(phi)/cos(theta)*q + cos(phi)/cos(theta)*r;
xdot(10) = (Iyy - Izz)*q*r/Ixx + L*T*sin(alpha)/Ixx;
xdot(11) = (Izz - Ixx)*p*r/Ixx - L*T*sin(beta)/Iyy;
xdot(12) = (Ixx - Iyy)*p*q/Izz + rcs(Izz);

end
